simulink model "understandingof_differentParametersOfWaves_UsingSinewave"  (R2024b)
settings: Solver=VariableStepDiscrete  StartTime=0.0  StopTime=inf  MaxStep=0.001  RelTol=1e-3
settings Model: PacingRate=0.100000  Creator=admin  LastModifiedBy=admin

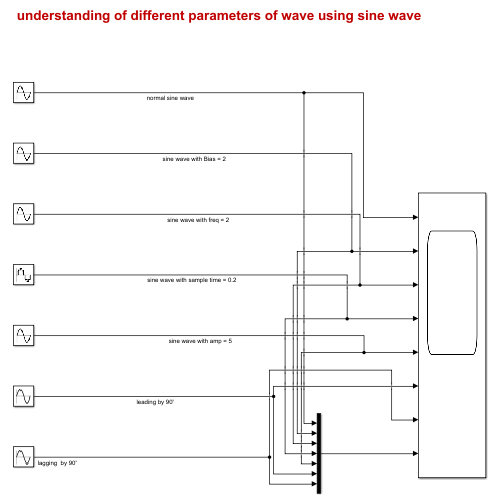
[thumbnail: Simulink's stored preview of the top-level diagram]
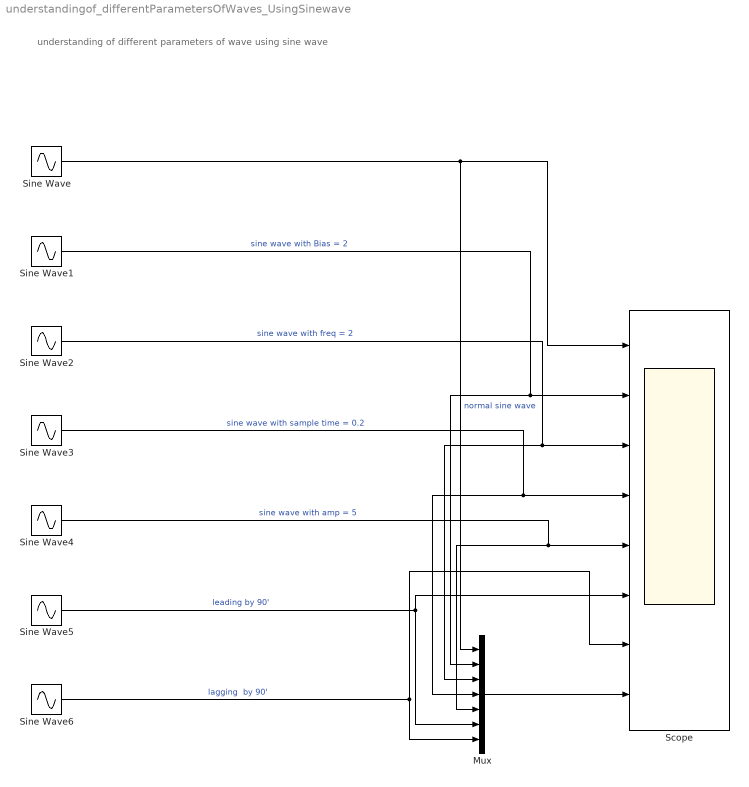
== system understandingof_differentParametersOfWaves_UsingSinewave ==
  note: understanding of different parameters of wave using sine wave
  Mux : Mux  Inputs=7
  Scope : Scope  NumInputPorts=8
  Sine Wave : Sin  SampleTime=0
  Sine Wave1 : Sin  Bias=2  SampleTime=0
  Sine Wave2 : Sin  Frequency=2  SampleTime=0
  Sine Wave3 : Sin  SampleTime=0.2
  Sine Wave4 : Sin  Amplitude=5  SampleTime=0
  Sine Wave5 : Sin  Phase=(pi/2)  SampleTime=0
  Sine Wave6 : Sin  Phase=-(pi/2)  SampleTime=0
  wires:
  Sine Wave/1 -> Scope/1, Mux/1  "normal sine wave"
  Sine Wave1/1 -> Scope/2, Mux/2  "sine wave with Bias = 2"
  Sine Wave2/1 -> Scope/3, Mux/3  "sine wave with freq = 2"
  Sine Wave3/1 -> Mux/4, Scope/4  "sine wave with sample time = 0.2"
  Sine Wave4/1 -> Scope/5, Mux/5  "sine wave with amp = 5"
  Sine Wave5/1 -> Mux/6, Scope/6  "leading by 90'"
  Sine Wave6/1 -> Scope/7, Mux/7  "lagging  by 90'"
  Mux/1 -> Scope/8
